simulink model "DDWMR"  (R2022a)
settings: Solver=FixedStepAuto  StartTime=0.0  StopTime=T_final  FixedStep=1e-3  MaxStep=1e-2  RelTol=1e-3
values from neighbouring files (symbols this model uses):
  BDD_thresh = 0.5    [Run_this_file_for_DDWMR_model.m]
  Cd = C    [Run_this_file_for_DDWMR_model.m]
  d = 0.1    [Dynamicfcn.m]    (also in Run_this_file_for_DDWMR_model.m; gps.m)
  I = 0.05    [Dynamicfcn.m]    (also in Run_this_file_for_DDWMR_model.m = 0.26903125)
  I_single = sort(randperm(n_meas,n_attack)).'    [Run_this_file_for_DDWMR_model.m]
  L = 0.235/2    (= 0.1175)    [Dynamicfcn.m]    (also in Run_this_file_for_DDWMR_model.m)
  m = 10    [Dynamicfcn.m]    (also in Run_this_file_for_DDWMR_model.m = 15)
  max_iter = 2000    [Run_this_file_for_DDWMR_model.m]
  q_initial = [theta0;x0;y0]    [Run_this_file_for_DDWMR_model.m]
  r = 0.05    [Dynamicfcn.m]    (also in Run_this_file_for_DDWMR_model.m)
  R = 1e-3    (= 0.001)    [Run_this_file_for_DDWMR_model.m]
  T_start_attack = .2*T_final    (= 4)    [Run_this_file_for_DDWMR_model.m]    (also in plot_results.m = .2*T_final)
  Ts = 0.01    [Dynamicfcn.m]    (also in Run_this_file_for_DDWMR_model.m; gps.m = 0.001; plot_results.m)
  V_initial = [v0;omega0]    [Run_this_file_for_DDWMR_model.m]
libraries: simulink x2, sharedTrackingLibrary x2
settings Model: Creator=yz19b  LastModifiedBy=Abely
settings SolverCC: AlgebraicLoopSolver=TrustRegion
settings DebuggingCC: UnconnectedInputMsg=warning  UnconnectedOutputMsg=warning  UnconnectedLineMsg=warning  SFMachineParentedDataDiag=warning

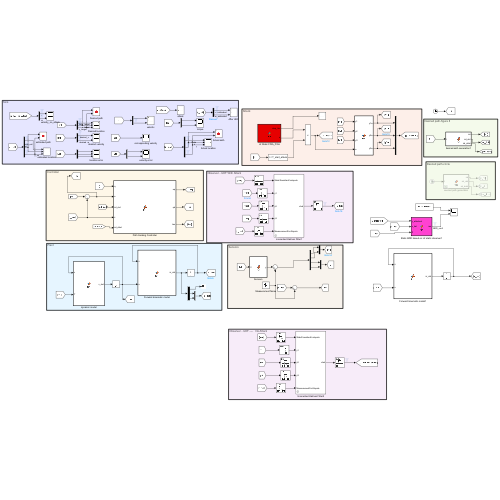
[thumbnail: Simulink's stored preview of the top-level diagram]
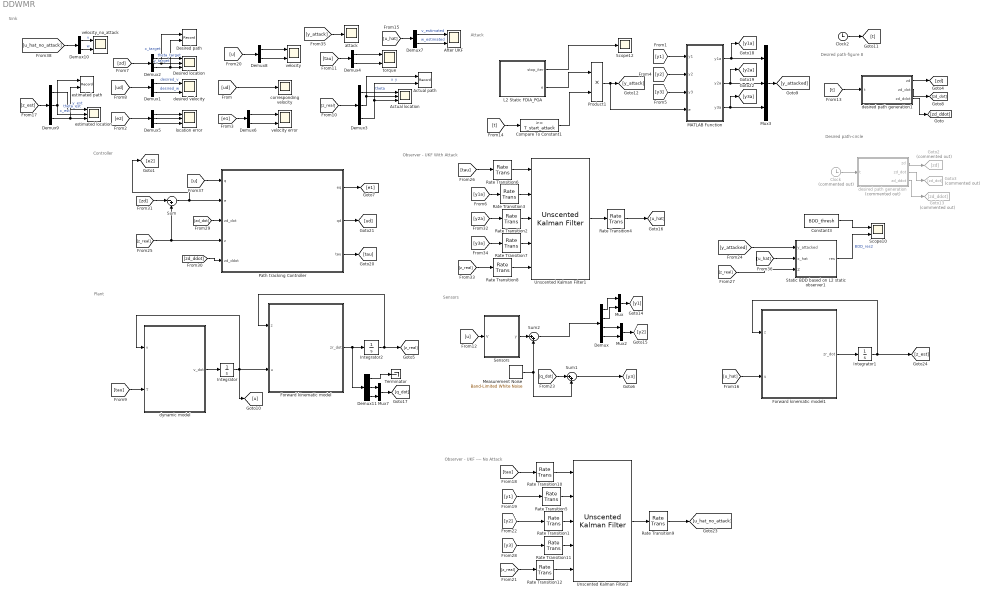
== system DDWMR ==
  note: Desired path-circle
  note: Sink
  note: Controller
  note: Plant
  note: Attack
  note: Observer - UKF With Attack
  note: Desired path-figure 8
  note: Sensors
  note: Observer - UKF ---- No Attack
  Actual location : Scope  NumInputPorts=3
  Actual path : Record  FileSettingsInternal="{\"entries\":[{\"content\":{\"excelSettings\":{\"content\":{},\"type\":\"Streamout.ExcelSettings\"}},\"type\":\"Streamout.FileSettingStorage\",\"uuid\":\"98e1b13d-32b0-4112-a3f4-17811f7e62ca\"}],\"packageUris\":[\"http://schema.mathworks.com/mf0/streamout_blocks/R2020a\"],\"version\":\"1.0\"}"  Layout=[1 1]  SignalsInternal="{\"entries\":[{\"content\":{\"signals\":[{\"content\":{\"blockPath\":[\"DDWMR_static/Actual path\"],\"channel\":[],\"dimensions\":[1],\"domain\":\"DDWMR_static/Actual path\",\"lineColor\":\"#a2142f\",\"plots\":[1],\"port\":1,\"sid\":[\"\"],\"signalID\":29295,\"signalName\":\"x\"},\"type\":\"RecordBlkView.Signal\",\"uuid\":\"77adc58b-3939-4672-9d1a-3a968cece15a\"},{\"content\":{\"blockPath\":[\"DDWMR_static/Actual path\"],\"channel\":[],\"dimensions\":[1],\"domain\":\"DDWMR_static/Actual path\",\"lineColor\":\"#139fff\",\"plots\":[1],\"port\":2,\"sid\":[\"\"],\"signalID\":29299,\"signalName\":\"y\"},\"type\":\"RecordBlkView.Signal\",\"uuid\":\"98d14323-1f21-416e-8de0-53ab9205d999\"}]},\"type\":\"RecordBlkView.InputSignals\",\"uuid\":\"623a91f1-7184-4913-9b76-83b9bfe60974\"}],\"packageUris\":[\"http://schema.mathworks.com/mf0/streamout_blocks/R2020a\"],\"version\":\"1.0\"}"  VisualizationBindings="{\"xyplotplugin\":{\"info\":[{\"series\":[{\"bindingParametersList\":[{\"parameter\":\"X-Axis\",\"signalID\":29295,\"signalName\":\"x\"},{\"parameter\":\"Y-Axis\",\"signalID\":29299,\"signalName\":\"y\"}],\"seriesID\":6406}],\"subplotID\":1}]}}"  CompatibilityTag=XY  st=-1
  After UKF : Scope  NumInputPorts=2
  Clock : Clock  Commented=on
  Clock2 : Clock
  Compare To Constant1 : simulink/Logic and Bit Operations/Compare To Constant  relop=>=  const=T_start_attack  OutDataTypeStr=boolean
  Constant3 : Constant  Value=BDD_thresh
  Demux : Demux
  Demux{1,4,6..8,10} (6 alike) : Demux  Outputs=2
  Demux{2..3,5,9,11} (5 alike) : Demux  Outputs=3
  Desired location : Scope  NumInputPorts=3
  "Desired path " : Record  FileSettingsInternal="{\"entries\":[{\"content\":{\"excelSettings\":{\"content\":{},\"type\":\"Streamout.ExcelSettings\"}},\"type\":\"Streamout.FileSettingStorage\",\"uuid\":\"f3e7e90d-5abe-44ea-bb83-89252e06a4a3\"}],\"packageUris\":[\"http://schema.mathworks.com/mf0/streamout_blocks/R2020a\"],\"version\":\"1.0\"}"  Layout=[1 1]  SignalsInternal="{\"entries\":[{\"content\":{\"signals\":[{\"content\":{\"blockPath\":[\"DDWMR_static/Desired path \"],\"channel\":[],\"dimensions\":[1],\"domain\":\"DDWMR_static/Desired path \",\"lineColor\":\"#a2142f\",\"plots\":[1],\"port\":1,\"sid\":[\"\"],\"signalID\":29303,\"signalName\":\"x_target\"},\"type\":\"RecordBlkView.Signal\",\"uuid\":\"e8263bb8-b269-4886-ad26-5befdf2ca8d7\"},{\"content\":{\"blockPath\":[\"DDWMR_static/Desired path \"],\"channel\":[],\"dimensions\":[1],\"domain\":\"DDWMR_static/Desired path \",\"lineColor\":\"#139fff\",\"plots\":[1],\"port\":2,\"sid\":[\"\"],\"signalID\":29307,\"signalName\":\"y_target\"},\"type\":\"RecordBlkView.Signal\",\"uuid\":\"a4db9f7a-11ad-4295-9363-4159a81bac38\"}]},\"type\":\"RecordBlkView.InputSignals\",\"uuid\":\"be5be972-1c84-4463-8d39-bd7b38efcc45\"}],\"packageUris\":[\"http://schema.mathworks.com/mf0/streamout_blocks/R2020a\"],\"version\":\"1.0\"}"  VisualizationBindings="{\"xyplotplugin\":{\"info\":[{\"series\":[{\"bindingParametersList\":[{\"parameter\":\"X-Axis\",\"signalID\":29303,\"signalName\":\"x_target\"},{\"parameter\":\"Y-Axis\",\"signalID\":29307,\"signalName\":\"y_target\"}],\"seriesID\":14060}],\"subplotID\":1}]}}"  CompatibilityTag=XY  st=-1
  Forward kinematic model : MATLAB Function  TreatAsAtomicUnit=on
  Forward kinematic model1 : MATLAB Function  TreatAsAtomicUnit=on
  Goto13 : Goto  Commented=on  GotoTag=zd_ddot
  Goto2 : Goto  Commented=on  GotoTag=zd
  Goto3 : Goto  Commented=on  GotoTag=zd_dot
  Integrator : Integrator  InitialCondition=V_initial
  Integrator1 : Integrator  InitialCondition=q_initial
  Integrator2 : Integrator  InitialCondition=q_initial
  L2 Static FDIA_PGA : MATLAB Function  TreatAsAtomicUnit=on
  MATLAB Function : MATLAB Function  TreatAsAtomicUnit=on
  Measurement Noise : simulink/Sources/Band-Limited White Noise  Cov=R*Ts  Ts=Ts  seed=[23341]
  Mux : Mux  Inputs=2
  Mux2 : Mux  Inputs=2
  Mux3 : Mux  Inputs=3
  Mux7 : Mux  Inputs=2
  Path tracking Controller : MATLAB Function  TreatAsAtomicUnit=on
  Product1 : Product
  Rate Transition{1..3,5..7,10..11} (8 alike) : RateTransition  InitialCondition=[0 0]  OutPortSampleTime=Ts
  Rate Transition12 : RateTransition  InitialCondition=[0 0 0]  OutPortSampleTime=Ts
  Rate Transition4 : RateTransition  Integrity=off  InitialCondition=1.6  OutPortSampleTime=0
  Rate Transition8 : RateTransition  InitialCondition=[0 0 0]  OutPortSampleTime=Ts
  Rate Transition9 : RateTransition  Integrity=off  InitialCondition=1.6  OutPortSampleTime=0
  Scope10 : Scope  NumInputPorts=2
  Scope12 : Scope
  Sensors : MATLAB Function  TreatAsAtomicUnit=on
  Static BDD based on L2 static observer1 : MATLAB Function  TreatAsAtomicUnit=on
  Sum : Sum  Inputs=|-+
  Sum1 : Sum  Inputs=|++
  Sum2 : Sum  Inputs=|++
  Terminator : Terminator
  Unscented Kalman Filter1 : sharedTrackingLibrary/Unscented Kalman Filter  StateTransitionFcn=Dynamicfcn  HasAdditiveProcessNoise=Additive  ProcessNoise=diag([1 1])  HasTimeVaryingProcessNoise=off  HasStateTransitionFcnExtraArgument=1  InitialState=[0 0]  InitialStateCovariance=1e-2  Alpha=1e-2  Beta=2  Kappa=0  MeasurementFcn1=gyroscope  HasMeasurementEnablePort1=off  HasAdditiveMeasurementNoise1=Additive  MeasurementNoise1=diag([R R])  HasTimeVaryingMeasurementNoise1=off  HasMeasurementFcnExtraArgument1=0  HasMeasurementWrapping1=off  MeasurementFcn2=encoder  HasMeasurementEnablePort2=off  HasAdditiveMeasurementNoise2=Additive  MeasurementNoise2=diag([R R])  HasTimeVaryingMeasurementNoise2=off  HasMeasurementFcnExtraArgument2=0  HasMeasurementWrapping2=off  MeasurementFcn3=gps  HasMeasurementEnablePort3=off  HasAdditiveMeasurementNoise3=Additive  MeasurementNoise3=diag([R R])  HasTimeVaryingMeasurementNoise3=off  HasMeasurementFcnExtraArgument3=1  HasMeasurementWrapping3=off  MeasurementFcn4=mfcn3  HasMeasurementEnablePort4=off  HasAdditiveMeasurementNoise4=Additive  MeasurementNoise4=R  HasTimeVaryingMeasurementNoise4=off  HasMeasurementFcnExtraArgument4=0  HasMeasurementWrapping4=off  MeasurementFcn5=myMeasurementFcn  HasMeasurementEnablePort5=off  HasAdditiveMeasurementNoise5=Additive  MeasurementNoise5=1  HasTimeVaryingMeasurementNoise5=off  HasMeasurementFcnExtraArgument5=0  HasMeasurementWrapping5=off  EnableMultirate=off  StateTransitionFcnSampleTime=1  MeasurementFcn1SampleTime=1  MeasurementFcn2SampleTime=1  MeasurementFcn3SampleTime=1  MeasurementFcn4SampleTime=1  MeasurementFcn5SampleTime=1  UseCurrentEstimator=on  OutputStateCovariance=off  DataType=double  SampleTime=Ts  NumberOfMeasurements=3
      settings: SourceProductBaseCode=TF,AE,PW,CT,DR,ID,LP,NV,AR,RO,RR,UV,VE
  Unscented Kalman Filter2 : sharedTrackingLibrary/Unscented Kalman Filter  StateTransitionFcn=Dynamicfcn  HasAdditiveProcessNoise=Additive  ProcessNoise=diag([1 1])  HasTimeVaryingProcessNoise=off  HasStateTransitionFcnExtraArgument=1  InitialState=[0 0]  InitialStateCovariance=1e-2  Alpha=1e-2  Beta=2  Kappa=0  MeasurementFcn1=gyroscope  HasMeasurementEnablePort1=off  HasAdditiveMeasurementNoise1=Additive  MeasurementNoise1=diag([R R])  HasTimeVaryingMeasurementNoise1=off  HasMeasurementFcnExtraArgument1=0  HasMeasurementWrapping1=off  MeasurementFcn2=encoder  HasMeasurementEnablePort2=off  HasAdditiveMeasurementNoise2=Additive  MeasurementNoise2=diag([R R])  HasTimeVaryingMeasurementNoise2=off  HasMeasurementFcnExtraArgument2=0  HasMeasurementWrapping2=off  MeasurementFcn3=gps  HasMeasurementEnablePort3=off  HasAdditiveMeasurementNoise3=Additive  MeasurementNoise3=diag([R R])  HasTimeVaryingMeasurementNoise3=off  HasMeasurementFcnExtraArgument3=1  HasMeasurementWrapping3=off  MeasurementFcn4=mfcn3  HasMeasurementEnablePort4=off  HasAdditiveMeasurementNoise4=Additive  MeasurementNoise4=R  HasTimeVaryingMeasurementNoise4=off  HasMeasurementFcnExtraArgument4=0  HasMeasurementWrapping4=off  MeasurementFcn5=myMeasurementFcn  HasMeasurementEnablePort5=off  HasAdditiveMeasurementNoise5=Additive  MeasurementNoise5=1  HasTimeVaryingMeasurementNoise5=off  HasMeasurementFcnExtraArgument5=0  HasMeasurementWrapping5=off  EnableMultirate=off  StateTransitionFcnSampleTime=1  MeasurementFcn1SampleTime=1  MeasurementFcn2SampleTime=1  MeasurementFcn3SampleTime=1  MeasurementFcn4SampleTime=1  MeasurementFcn5SampleTime=1  UseCurrentEstimator=on  OutputStateCovariance=off  DataType=double  SampleTime=Ts  NumberOfMeasurements=3
      settings: SourceProductBaseCode=TF,AE,PW,CT,DR,ID,LP,NV,AR,RO,RR,UV,VE
  attack : Scope
  corresponding velocity : Scope
  desired path generation : MATLAB Function  Commented=on  TreatAsAtomicUnit=on
  desired path generation1 : MATLAB Function  TreatAsAtomicUnit=on
  desired velocity : Scope  NumInputPorts=2
  dynamic model : MATLAB Function  TreatAsAtomicUnit=on
  estimated location : Scope  NumInputPorts=3
  estimated path : Record  FileSettingsInternal="{\"entries\":[{\"content\":{\"excelSettings\":{\"content\":{},\"type\":\"Streamout.ExcelSettings\"}},\"type\":\"Streamout.FileSettingStorage\",\"uuid\":\"3e4c8b0d-3d69-40b4-8e60-ca6d524e3c1c\"}],\"packageUris\":[\"http://schema.mathworks.com/mf0/streamout_blocks/R2020a\"],\"version\":\"1.0\"}"  Layout=[1 1]  SignalsInternal="{\"entries\":[{\"content\":{\"signals\":[{\"content\":{\"blockPath\":[\"DDWMR_static/estimated path\"],\"channel\":[],\"dimensions\":[1],\"domain\":\"DDWMR_static/estimated path\",\"lineColor\":\"#ff13a6\",\"plots\":[],\"port\":1,\"sid\":[\"\"],\"signalID\":29389,\"signalName\":\"x_est\"},\"type\":\"RecordBlkView.Signal\",\"uuid\":\"b1e6ec60-7eb2-4e81-8cbf-b7fb0dc4cbaa\"},{\"content\":{\"blockPath\":[\"DDWMR_static/estimated path\"],\"channel\":[],\"dimensions\":[1],\"domain\":\"DDWMR_static/estimated path\",\"lineColor\":\"#fe330a\",\"plots\":[],\"port\":2,\"sid\":[\"\"],\"signalID\":29393,\"signalName\":\"y_est\"},\"type\":\"RecordBlkView.Signal\",\"uuid\":\"7038b5bf-4498-4102-9773-92d52c2aed0b\"}]},\"type\":\"RecordBlkView.InputSignals\",\"uuid\":\"f984c6d8-4562-4a4d-a3e6-e33bab7189a5\"}],\"packageUris\":[\"http://schema.mathworks.com/mf0/streamout_blocks/R2020a\"],\"version\":\"1.0\"}"  VisualizationBindings="{\"xyplotplugin\":{\"info\":[{\"series\":[],\"subplotID\":1}]}}"  CompatibilityTag=XY  st=-1
  location error : Scope  NumInputPorts=3
  torque : Scope  NumInputPorts=2
  velocity : Scope  NumInputPorts=2
  velocity error : Scope  NumInputPorts=2
  velocity_no_attack : Scope  NumInputPorts=2
  wires:
  Clock/1 -> desired path generation/1(t)
  [ud] -> Demux1/1
  Demux1/1 -> desired velocity/1  "desired_v"
  Demux1/2 -> desired velocity/2  "desired_w"
  desired path generation/2(zd_dot) -> Goto3/1
  desired path generation/1(zd) -> Goto2/1
  [zd] -> Demux2/1
  Demux2/1 -> Desired location/1  "theta_target"
  Demux2/2 -> "Desired path "/1, Desired location/2  "x_target"
  Demux2/3 -> "Desired path "/2, Desired location/3  "y_target"
  [tau] -> dynamic model/2(T)
  Forward kinematic model/1(zr_dot) -> Demux11/1, Integrator2/1
  Integrator2/1 -> [z_real], Forward kinematic model/1(z)
  [z_real] -> Demux3/1
  Demux3/3 -> Actual path/2, Actual location/3  "y"
  Demux3/2 -> Actual path/1, Actual location/2  "x"
  Demux3/1 -> Actual location/1  "theta"
  Demux4/2 -> torque/2
  Demux4/1 -> torque/1
  [tau] -> Demux4/1
  [e2] -> Demux5/1
  Demux5/1 -> location error/1
  Demux5/2 -> location error/2
  Demux6/2 -> velocity error/2
  Demux6/1 -> velocity error/1
  [e1] -> Demux6/1
  dynamic model/1(v_dot) -> Integrator/1
  [ud] -> corresponding velocity/1
  [u] -> Sensors/1(V)
  Sensors/1(y) -> Sum2/1
  Sum1/1 -> [y3]
  Sum2/1 -> Demux/1
  Demux/1 -> Mux/1
  Demux/2 -> Mux/2
  Demux/3 -> Mux2/1
  Demux/4 -> Mux2/2
  Mux/1 -> [y1]
  Mux2/1 -> [y2]
  [q_dot] -> Sum1/1
  Measurement Noise/1 -> Sum1/2, Sum2/2
  Demux7/1 -> After UKF/1  "v_estimated"
  Demux7/2 -> After UKF/2  "w_estimated"
  [u_hat] -> Demux7/1
  Integrator/1 -> Forward kinematic model/2(u), dynamic model/1(v), [u]
  Rate Transition4/1 -> [u_hat]
  [tau] -> Rate Transition6/1
  Unscented Kalman Filter1/1 -> Rate Transition4/1
  Rate Transition6/1 -> Unscented Kalman Filter1/1
  Demux11/2 -> Mux7/1
  Demux11/3 -> Mux7/2
  Mux7/1 -> [q_dot]
  Demux11/1 -> Terminator/1
  [z_real] -> Rate Transition8/1
  Rate Transition8/1 -> Unscented Kalman Filter1/5
  desired path generation1/1(zd) -> [zd]
  desired path generation1/2(zd_dot) -> [zd_dot]
  [t] -> desired path generation1/1(t)
  desired path generation/3(zd_ddot) -> Goto13/1
  [z_real] -> Sum/2, Path tracking Controller/4(z)
  [zd_dot] -> Path tracking Controller/3(zd_dot)
  [zd_ddot] -> Path tracking Controller/5(zd_ddot)
  [zd] -> Sum/1
  Sum/1 -> [e2], Path tracking Controller/2(e)
  Path tracking Controller/3(tau) -> [tau]
  Path tracking Controller/2(qd) -> [ud]
  desired path generation1/3(zd_ddot) -> [zd_ddot]
  Demux5/3 -> location error/3
  Path tracking Controller/1(eq) -> [e1]
  [u] -> Path tracking Controller/1(q)
  Clock2/1 -> [t]
  L2 Static FDIA_PGA/1(stop_iter) -> Scope12/1
  [t] -> Compare To Constant1/1
  Compare To Constant1/1 -> Product1/2
  L2 Static FDIA_PGA/2(e) -> Product1/1
  [u_hat] -> Static BDD based on L2 static observer1/2(x_hat)
  Static BDD based on L2 static observer1/1(res) -> Scope10/2  "BDD_res2"
  [y_attacked] -> Static BDD based on L2 static observer1/1(y_attacked)
  Constant3/1 -> Scope10/1
  [y3] -> MATLAB Function/3(y3)
  [y1] -> MATLAB Function/1(y1)
  Product1/1 -> MATLAB Function/4(e), [y_attack]
  [y2] -> MATLAB Function/2(y2)
  MATLAB Function/2(y2a) -> Mux3/2, [y2a]
  MATLAB Function/3(y3a) -> Mux3/3, [y3a]
  Mux3/1 -> [y_attacked]
  [y1a] -> Rate Transition3/1
  [y2a] -> Rate Transition2/1
  [y3a] -> Rate Transition7/1
  [y_attack] -> attack/1
  Rate Transition3/1 -> Unscented Kalman Filter1/2
  Rate Transition2/1 -> Unscented Kalman Filter1/3
  Rate Transition7/1 -> Unscented Kalman Filter1/4
  MATLAB Function/1(y1a) -> [y1a], Mux3/1
  [z_real] -> Static BDD based on L2 static observer1/3(Z)
  Forward kinematic model1/1(zr_dot) -> Integrator1/1
  Integrator1/1 -> [z_est], Forward kinematic model1/1(z)
  [u_hat] -> Forward kinematic model1/2(u)
  Demux9/2 -> estimated path/1, estimated location/2  "x_est"
  Demux9/3 -> estimated path/2, estimated location/3  "y_est"
  Demux9/1 -> estimated location/1  "theta_est"
  [z_est] -> Demux9/1
  Rate Transition1/1 -> Unscented Kalman Filter2/3
  Rate Transition5/1 -> Unscented Kalman Filter2/2
  Rate Transition11/1 -> Unscented Kalman Filter2/4
  [y2] -> Rate Transition1/1
  Unscented Kalman Filter2/1 -> Rate Transition9/1
  Rate Transition10/1 -> Unscented Kalman Filter2/1
  Rate Transition9/1 -> [u_hat_no_attack]
  [z_real] -> Rate Transition12/1
  [tau] -> Rate Transition10/1
  Rate Transition12/1 -> Unscented Kalman Filter2/5
  [y1] -> Rate Transition5/1
  [y3] -> Rate Transition11/1
  Demux10/1 -> velocity_no_attack/1  "v"
  Demux10/2 -> velocity_no_attack/2  "w"
  [u_hat_no_attack] -> Demux10/1
  [u] -> Demux8/1
  Demux8/1 -> velocity/1
  Demux8/2 -> velocity/2

== matlab function DDWMR/desired path generation ==
  data: t input; zd output; zd_dot output; zd_ddot output
function [zd,zd_dot,zd_ddot] = fcn(t)


% unit circle (radius = 1; origin: (0,0))
zd = [t;
      cos(t);         % x
      sin(t)];        % y

zd_dot = [-sin(t);
          cos(t)];
      
zd_ddot = [-cos(t);
           -sin(t)];

== matlab function DDWMR/Static BDD based on L2 static observer1 ==
  data: y_attacked input; x_hat input; res output; Z input; r parameter; L parameter; d parameter
function res = fcn(y_attacked,x_hat,Z, r, L, d)

theta = Z(1);
C = [1, 0;
    0, 1;
    0.25/r,0.25*L/r;
    0.25/r,-0.25*L/r;
    cos(theta),-d*sin(theta);
    sin(theta),d*cos(theta)];

res = norm(y_attacked-C*x_hat,2);

== matlab function DDWMR/desired path generation1 ==
  data: t input; zd output; zd_dot output; zd_ddot output
function [zd,zd_dot,zd_ddot] = fcn(t)

a=1;
x = a*cos(t)/(1+sin(t)^2);
y = a*sin(t)*cos(t)/(1+sin(t)^2);
% unit circle (radius = 1; origin: (0,0))
zd = [atan(y./x);              % theta
      a*cos(t)/(1+sin(t)^2);         % x
      a*sin(t)*cos(t)/(1+sin(t)^2)];        % y

zd_dot = [-a*sin(t)*(cos(t)^2+2)/(1+sin(t)^2)^2;
          (a*cos(t)^2-2*a*sin(t)^2)/(1+sin(t)^2)^2];

z1 = (a*sin(t)^2*cos(t)^3-11*a*cos(t)^3+8*a*cos(t))/(1+sin(t)^2)^3;
z2 = -2*a*sin(t)*cos(t)*(3+2*cos(t)^2-sin(t)^2)/(1+sin(t)^2)^3;
zd_ddot = [z1;
           z2];

== matlab function DDWMR/Forward kinematic model1 ==
  data: z input; u input; zr_dot output; d parameter; r parameter
function zr_dot = fcn(z,u,d,r)

%% unpacking the state vectors
theta=z(1);

%% unpacking the intput
v=u(1);
omega=u(2);

%% ODE
theta_dot=omega;
x_dot=v*cos(theta)-d*omega*sin(theta);
y_dot=v*sin(theta)+d*omega*cos(theta);
% phir_dot = (v+omega)/r;
% phil_dot = (v-omega)/r;


%% packing the output
zr_dot=[theta_dot;x_dot;y_dot];

== matlab function DDWMR/MATLAB Function ==
  data: y1 input; y1a output; y2 input; y3 input; e input; y2a output; y3a output
function [y1a,y2a,y3a] = fcn(y1,y2,y3,e)

y1_size = length(y1);
y2_size = length(y2);
% y3_size = length(y3);

y1a = y1 + e(1:y1_size);
y2a = y2 + e(y1_size+1:y1_size+y2_size);
y3a = y3 + e(y1_size+y2_size+1:end);

== matlab function DDWMR/Sensors ==
  data: V input; y output; r parameter; L parameter
function y = fcn(V,r,L)

C=[1,0;
    0,1;
    1/(4*r),L/(4*r);
    1/(4*r),-L/(4*r)];
y=C*V;

== matlab function DDWMR/Path tracking Controller ==
  data: eq output; qd output; q input; tau output; e input; zd_dot input; z input; zd_ddot input; m parameter; d parameter; r parameter; L parameter; I parameter
function [eq,qd,tau] = fcn(q,e,zd_dot,z,zd_ddot,m, d, r, L, I)


kq =15;
ke =15;
ez = e(2:3);
% e_theta = e(1);
theta = z(1);
omega = q(2);

B_inver=-(r/(2*L))*[-L,-1;-L,1];
M=[m,0;
    0,m*d*d+I];
D=[0,-m*d*omega;
    m*d*omega,0];
C = [cos(theta), -d*sin(theta);
     sin(theta), d*cos(theta)];
C_bar_tran = [0, cos(theta), sin(theta);
              1, -d*sin(theta), d*cos(theta)];
C_inver = (1/d)*[d*cos(theta), d*sin(theta);
                 -sin(theta), cos(theta)];
C_inver_dot = (1/d)*[-d*sin(theta)*omega, d*cos(theta)*omega;
                     -cos(theta)*omega, -sin(theta)*omega];


qd = C_inver*(zd_dot-ke*ez);
qd_dot = -ke*(C_inver_dot*ez+q)+C_inver*(zd_ddot+ke*zd_dot+C*C_inver_dot*zd_dot);
u = -kq*(q-qd)+qd_dot-C_bar_tran*e;
tau = B_inver*(M*u+D*q);
eq = q-qd;

== matlab function DDWMR/Forward kinematic model ==
  data: z input; u input; zr_dot output; d parameter; r parameter
function zr_dot = fcn(z,u,d,r)

%% unpacking the state vectors
theta=z(1);

%% unpacking the intput
v=u(1);
omega=u(2);

%% ODE
theta_dot=omega;
x_dot=v*cos(theta)-d*omega*sin(theta);
y_dot=v*sin(theta)+d*omega*cos(theta);
% phir_dot = (v+omega)/r;
% phil_dot = (v-omega)/r;


%% packing the output
zr_dot=[theta_dot;x_dot;y_dot];

== matlab function DDWMR/dynamic model ==
  data: v_dot output; v input; T input; L parameter; r parameter; d parameter; m parameter; I parameter
function v_dot = fcn(v, T,L, r, d, m,I)

%% unpacking intput
omega=v(2);

%% Parameter
M_temp=[m*d*d+I,0;
         0,m];

M_inver=(1/(m*(m*d*d+I)))*M_temp;

D=[0,-m*d*omega;
    m*d*omega,0];

B=(1/r)*[1,1;L,-L];

%% ODE
v_dot=M_inver*(-D*v+B*T);

== matlab function DDWMR/L2 Static FDIA_PGA ==
  data: stop_iter output; I_single parameter; e output; Cd parameter; BDD_thresh parameter; max_iter parameter
function [stop_iter,e]  = fcn(I_single,Cd, BDD_thresh,max_iter)

%% Measurement Channel Attack
%  Assumptions:
%  1. The attacker knows the actual measurement
%  2. The attacker can only corrupt upto n_attack measurements
%  3. The attacker knows the BDD theshold

attack_idx = I_single;
% e = L2_FDIA(C_obsv_d,attack_idx,0.9*BDD_thresh);

[stop_iter,e] = L2_FDIA2(Cd,attack_idx,BDD_thresh,max_iter);
